simulink model "Project_LeadControllerLimiter"  (R2020a)
settings: Solver=ode15s  StartTime=0.0  StopTime=20  RelTol=1e-3
undefined symbols (not defined in the file or in its folder): i_ss, m, y_ss
settings Model: Creator=Joey Baby  LastModifiedBy=Joey Baby

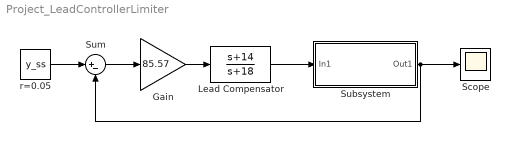
== system Project_LeadControllerLimiter ==
  Gain : Gain  Gain=85.57
  Lead Compensator : TransferFcn  Numerator=[1 14]  Denominator=[1 18]
  Scope : Scope
  Subsystem : Subsystem
  Sum : Sum  Inputs=|+-
  r=0.05 : Constant  Value=y_ss
  wires:
  Gain/1 -> Lead Compensator/1
  Lead Compensator/1 -> Subsystem/1(In1)
  r=0.05/1 -> Sum/1
  Sum/1 -> Gain/1
  Subsystem/1(Out1) -> Sum/2, Scope/1

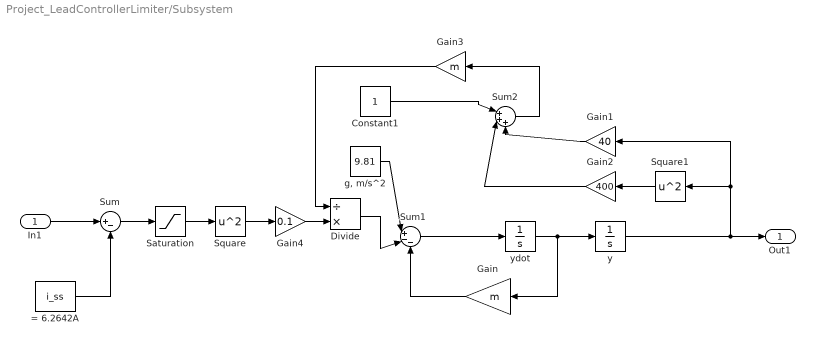
== system Project_LeadControllerLimiter/Subsystem ==
  In1 : Inport
  = 6.2642A : Constant  Value=i_ss
  Constant1 : Constant
  Divide : Product  Inputs=/*
  Gain : Gain  Gain=m
  Gain1 : Gain  Gain=40
  Gain2 : Gain  Gain=400
  Gain3 : Gain  Gain=m
  Gain4 : Gain  Gain=0.1
  Saturation : Saturate  UpperLimit=15  LowerLimit=-15
  Square : Math  Operator=square  SaturateOnIntegerOverflow=on
  Square1 : Math  Operator=square  SaturateOnIntegerOverflow=on
  Sum : Sum  Inputs=|+-
  Sum1 : Sum  Inputs=|+--
  Sum2 : Sum  Inputs=|+++
  "g, m/s^2" : Constant  Value=9.81
  y : Integrator  InitialCondition=0.05
  ydot : Integrator  InitialCondition=0.01
  Out1 : Outport
  wires:
  Gain3/1 -> Divide/1
  Saturation/1 -> Square/1
  Sum/1 -> Saturation/1
  Sum1/1 -> ydot/1
  Gain2/1 -> Sum2/2
  = 6.2642A/1 -> Sum/2
  Divide/1 -> Sum1/2
  y/1 -> Square1/1, Gain1/1, Out1/1
  "g, m/s^2"/1 -> Sum1/1
  Gain/1 -> Sum1/3
  ydot/1 -> Gain/1, y/1
  Sum2/1 -> Gain3/1
  In1/1 -> Sum/1
  Square1/1 -> Gain2/1
  Gain1/1 -> Sum2/3
  Square/1 -> Gain4/1
  Gain4/1 -> Divide/2
  Constant1/1 -> Sum2/1
